simulink model "Inverter3ph__lca_SPS"  (Simulink 8.4)
settings: Solver=FixedStepDiscrete  StartTime=0.0  StopTime=0.1  FixedStep=Ts  RelTol=1e-3
PreLoadFcn:
  | Ts=20e-6
InitFcn:
  | Ts=20e-6
libraries: powerlib x12
settings Model: Creator=AlirezaJavadi  LastModifiedBy=OPAL-RT  BufferReuse=off
settings SolverCC: AutoInsertRateTranBlk=on
settings OptimizationCC: BlockReduction=off  OptimizeBlockIOStorage=off  BufferReuse=off  GlobalBufferReuse=off  ExpressionFolding=off  LocalBlockOutputs=off
settings DebuggingCC: FcnCallInpInsideContextMsg=EnableAllAsWarning

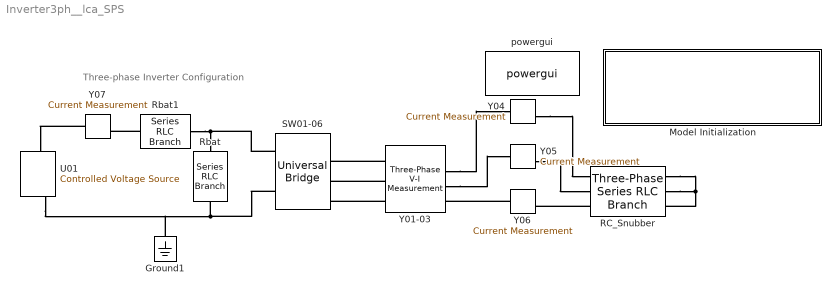
== system Inverter3ph__lca_SPS ==
  note: Three-phase Inverter Configuration
  Ground1 : powerlib/Elements/Ground  LConnTagsString=a
  Model Initialization : Subsystem  mask(Model Initialization, (A.J)){Ts=Ts=20e-6}
      mask prompts: Ts "Fixed Sample time-step size (s)"
      mask help:
      | 1- Choose Fixed-step in the Solver options.
      | 2- Write “Ts” as Fixed-step size.
      | 3- Choose MultiTasking and Automatically handle rate transition.
      | Finally enter the discrete Step-time for simulation here.
      mask init:
      | Block = gcb;
      | Name = bdroot(Block);
      | pos = get_param(Block, 'Position');
      | height = pos(4) - pos(2);
      | set_param(Name, 'PreLoadFcn', Ts);
      | set_param(Name, 'InitFcn', Ts);
      | infor = ['  ', upper(Name), '\n  ', get_param(Name, 'InitFcn') ' (s)', '\n\n ', date];
      mask Display: text(0.5, height*0.5, infor, 'horizontalAlignment', 'left', 'verticalAlignment', 'middle') ;
  RC_Snubber : powerlib/Elements/Three-Phase Series RLC Branch  LConnTagsString=A|B|C  RConnTagsString=A|B|C  BranchType=RL  Resistance=50e-3  Inductance=1e-3  Capacitance=1e-6  Measurements=None
  Rbat : powerlib/Elements/Series RLC Branch  LConnTagsString=__new0  RConnTagsString=__new0  BranchType=R  Resistance=10000  Inductance=1e-3  SetiL0=off  InitialCurrent=0  Capacitance=1e-6  Setx0=off  InitialVoltage=0  Measurements=None
  Rbat1 : powerlib/Elements/Series RLC Branch  LConnTagsString=__new0  RConnTagsString=__new0  BranchType=R  Resistance=1e-3  Inductance=1e-3  SetiL0=off  InitialCurrent=0  Capacitance=1e-6  Setx0=off  InitialVoltage=0  Measurements=None
  SW01-06 : powerlib/Power Electronics/Universal Bridge  Arms=3  SnubberResistance=1e5  SnubberCapacitance=inf  Device=IGBT / Diodes  Ron=1e-3  Lon=0  ForwardVoltages="[  0  0  ]"  ForwardVoltage=0  GTOparameters=[ 10e-6 , 20e-6 ]  IGBTparameters=[ 1e-6 , 2e-6 ]  Measurements=None  Measurements_2=None  converterType=Rectifier
  "U01 " : powerlib/Electrical Sources/Controlled Voltage Source  Initialize=on  Source_Type=AC  Amplitude=0  Phase=0  Frequency=0  Measurements=None
  Y01-03 : powerlib/Measurements/Three-Phase V-I Measurement  VoltageMeasurement=phase-to-ground  SetLabelV=off  LabelV=Vabc  Vpu=off  VpuLL=off  CurrentMeasurement=no  SetLabelI=off  LabelI=Iabc  Ipu=off  Pbase=100e6  Vbase=500e3  OutputType=Complex  PhasorSimulation=off  PSBequivalent=0
  Y04 : powerlib/Measurements/Current Measurement  PhasorSimulation=off  OutputType=Complex  PSBequivalent=0
  Y05 : powerlib/Measurements/Current Measurement  PhasorSimulation=off  OutputType=Complex  PSBequivalent=0
  Y06 : powerlib/Measurements/Current Measurement  PhasorSimulation=off  OutputType=Complex  PSBequivalent=0
  "Y07 " : powerlib/Measurements/Current Measurement  PhasorSimulation=off  OutputType=Complex  PSBequivalent=0
  powergui : powerlib/powergui  SimulationMode=Discrete  SolverType=Tustin  SampleTime=Ts  frequency=60  SPID=off  DisableSnubberDevices=off  DisableRonSwitches=off  DisableVfSwitches=off  SwTol=0  DisplayEquations=off  Interpol=off  methode=off  Ts=0  frequencyindice=0  Pbase=100e6  ErrMax=1e-4  Iterations=50  UnitsV=kV  UnitsW=MW  FunctionMessages=off  echomessages=off  HookPort=off  EnableUseOfTLC=off  x0status=blocks  RestoreLinks=warning  ResistiveCurrentMeasurement=off  Frange=[0:2:500]  Ylog=off  Xlog=on  ShowGrid=off  save=off  variable=ZData  structure=sps1phPWM1_str  ZoomFFT=on  StartTime=0.1-2/60  cycles=2  DisplayStyle=1  fundamental=60  FreqAxis=off  MaxFrequency=5000  frequencyindicesteady=1  RmsSteady=1  display=off
  connections:
  "Y07 "/LConn1 -- "U01 "/RConn1
  Y01-03/RConn1 -- Y04/LConn1
  Y01-03/LConn3 -- SW01-06/LConn3
  Y01-03/LConn2 -- SW01-06/LConn2
  Y01-03/LConn1 -- SW01-06/LConn1
  Y01-03/RConn2 -- Y05/LConn1
  RC_Snubber/LConn3 -- Y06/RConn1
  RC_Snubber/RConn2 -- RC_Snubber/RConn3 -- RC_Snubber/RConn1
  Y04/RConn1 -- RC_Snubber/LConn1
  Y05/RConn1 -- RC_Snubber/LConn2
  Y06/LConn1 -- Y01-03/RConn3
  Rbat1/RConn1 -- "Y07 "/RConn1
  Rbat1/LConn1 -- Rbat/LConn1 -- SW01-06/RConn1
  SW01-06/RConn2 -- Ground1/LConn1 -- "U01 "/LConn1 -- Rbat/RConn1

== system Inverter3ph__lca_SPS/Model Initialization ==
